simulink model "longitudinalMotion"  (R2023b)
settings: Solver=VariableStepAuto  StartTime=0.0  StopTime=30  FixedStep=0.01  RelTol=1e-3  AbsTol=1e-3  EnableMultiTasking=on
PreLoadFcn:
  | load terrainData
  | vehicleData
undefined symbols (not defined in the file or in its folder): FL, FR, RL, RR, slope
libraries: fl_lib x5, nesl_utility x4, sdl_lib x4, chassisTires_lib x1
settings Model: Creator=sseshadr  LastModifiedBy=mmedi
settings SolverCC: AutoScaleAbsTol=off  AlgebraicLoopSolver=TrustRegion
settings DataIOCC: LimitDataPoints=on  SaveFormat=Array  ReturnWorkspaceOutputs=off  SignalLoggingName=logsout_longitudinalMotion
settings OptimizationCC: ReuseModelBlockBuffer=off  LifeSpan=inf
settings DebuggingCC: UnconnectedInputMsg=warning  UnconnectedOutputMsg=warning  UnconnectedLineMsg=warning  SFUnexpectedBacktrackingDiag=warning  SFNoUnconditionalDefaultTransitionDiag=warning  SFExecutionAtInitializationDiag=none  ArithmeticOperatorsInVariantConditions=warning
settings HardwareCC: ProdBitPerPointer=32  ProdBitPerSizeT=32  ProdBitPerPtrDiffT=32  ProdLargestAtomicFloat=None  ProdIntDivRoundTo=Undefined  ProdEndianess=Unspecified  ProdWordSize=32  ProdHWDeviceType=32-bit Generic
settings ModelReferenceCC: EnableRefExpFcnMdlSchedulingChecks=on  PropagateSignalLabelsOutOfModel=off
settings SFSimCC: SimUseLocalCustomCode=off  CustomCodeUndefinedFunction=UseInterfaceOnly
settings RTWCC: RTWUseLocalCustomCode=off
settings CodeAppCC: StateflowObjectComments=on
settings GRTTargetCC: TargetLangStandard=C89/C90 (ANSI)
settings ConfigComp: CovMetricSettings=dw  CovSaveCumulativeToWorkspaceVar=on  CovSaveSingleToWorkspaceVar=on  CovExternalEMLEnable=off
settings SimscapeCC: SimscapeNormalizeSystem=off  SimscapeLogType=all  SimscapeLogSimulationStatistics=on  SimscapeLogToSDI=on  SimscapeLogName=simlog_longitudinalMotion  SimscapeLogDataHistory=10000

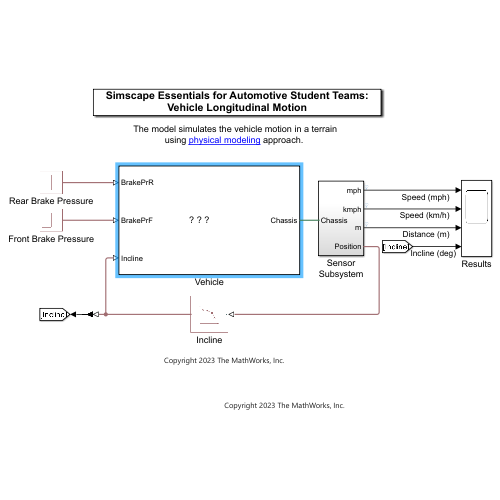
[thumbnail: Simulink's stored preview of the top-level diagram]
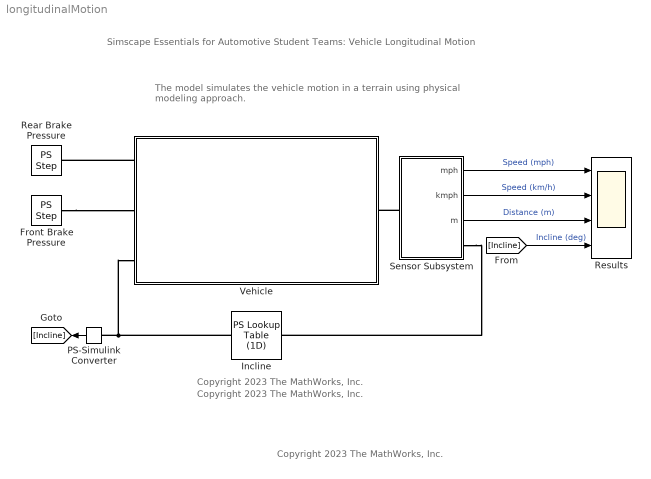
== system longitudinalMotion ==
  note: Copyright 2023 The MathWorks, Inc.
  note: Simscape Essentials for Automotive Student Teams: Vehicle Longitudinal Motion
  note: The model simulates the vehicle motion in a terrain using physical modeling approach.
  note: Copyright 2023 The MathWorks, Inc.
  note: Copyright 2023 The MathWorks, Inc.
  Front Brake Pressure : fl_lib/Physical Signals/Sources/PS Step  step_time=15 s  initial_value=0 N/m^2  final_value=brake.frontPressure N/(m^2)
  Incline : fl_lib/Physical Signals/Lookup Tables/PS Lookup Table (1D)  x=dist m  f=slope*1.2 rad  interp_method=simscape.enum.interpolation.linear  extrap_method=simscape.enum.extrapolation.linear
  PS-Simulink Converter : nesl_utility/PS-Simulink Converter  PhysicalDomain=network_engine_domain  SubClassName=ps_output  LeftPortType=input  RightPortType=output  PseudoPeriodic=off  Frequencies=[]  VectorFormat=inherit  Unit=deg  AffineConversion=off
  Rear Brake Pressure : fl_lib/Physical Signals/Sources/PS Step  step_time=12 s  initial_value=0 N/m^2  final_value=brake.rearPressure N/(m^2)
  Results : Scope  NumInputPorts=4
  Sensor Subsystem : Subsystem
  Vehicle : Subsystem
      mask Display: image('Images/vehicle.jpg'); % Use "Edit Image" on toolstrip to change.
  wires:
  Sensor Subsystem/1(mph) -> Results/1  "Speed (mph)"
  Sensor Subsystem/2(kmph) -> Results/2  "Speed (km/h)"
  Sensor Subsystem/3(m) -> Results/3  "Distance (m)"
  PS-Simulink Converter/1 -> [Incline]
  [Incline] -> Results/4  "Incline (deg)"
  connections:
  Sensor Subsystem/LConn1 -- Vehicle/RConn1
  Incline/RConn1 -- Vehicle/LConn3 -- PS-Simulink Converter/LConn1
  Sensor Subsystem/RConn1 -- Incline/LConn1
  Vehicle/LConn1 -- Rear Brake Pressure/RConn1
  Front Brake Pressure/RConn1 -- Vehicle/LConn2

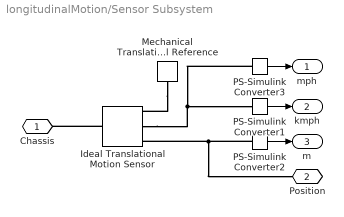
== system longitudinalMotion/Sensor Subsystem ==
  Ideal Translational Motion Sensor : fl_lib/Mechanical/Mechanical Sensors/Ideal Translational Motion Sensor  reference=foundation.enum.MeasurementReference.difference  acceleration_port=false  velocity_port=true  position_port=true  offset=0 m
  Mechanical Translational Reference : fl_lib/Mechanical/Translational Elements/Mechanical Translational Reference
  PS-Simulink Converter1 : nesl_utility/PS-Simulink Converter  PhysicalDomain=network_engine_domain  SubClassName=ps_output  LeftPortType=input  RightPortType=output  PseudoPeriodic=off  Frequencies=[]  VectorFormat=1-D array  Unit=km/hr  AffineConversion=off
  PS-Simulink Converter2 : nesl_utility/PS-Simulink Converter  PhysicalDomain=network_engine_domain  SubClassName=ps_output  LeftPortType=input  RightPortType=output  PseudoPeriodic=off  Frequencies=[]  VectorFormat=1-D array  Unit=1  AffineConversion=off
  PS-Simulink Converter3 : nesl_utility/PS-Simulink Converter  PhysicalDomain=network_engine_domain  SubClassName=ps_output  LeftPortType=input  RightPortType=output  PseudoPeriodic=off  Frequencies=[]  VectorFormat=1-D array  Unit=mph  AffineConversion=off
  Chassis : PMIOPort  Side=Left
  Position : PMIOPort  Port=2  Side=Right
  mph : Outport  VectorParamsAs1DForOutWhenUnconnected=off
  kmph : Outport  Port=2  VectorParamsAs1DForOutWhenUnconnected=off
  m : Outport  Port=3  VectorParamsAs1DForOutWhenUnconnected=off
  wires:
  PS-Simulink Converter1/1 -> kmph/1
  PS-Simulink Converter2/1 -> m/1
  PS-Simulink Converter3/1 -> mph/1
  connections:
  Mechanical Translational Reference/LConn1 -- Ideal Translational Motion Sensor/RConn1
  PS-Simulink Converter2/LConn1 -- Position/RConn1 -- Ideal Translational Motion Sensor/RConn3
  Ideal Translational Motion Sensor/RConn2 -- PS-Simulink Converter1/LConn1 -- PS-Simulink Converter3/LConn1
  Ideal Translational Motion Sensor/LConn1 -- Chassis/RConn1

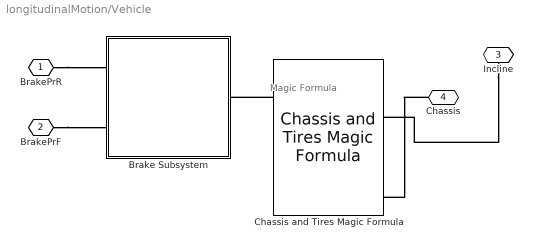
== system longitudinalMotion/Vehicle ==
  note: Magic Formula
  Brake Subsystem : Subsystem
  Chassis and Tires Magic Formula : chassisTires_lib/Chassis and Tires Magic Formula  SystemSampleTime=-1  VariantActivationTime=update diagram  AllowFlexibleInterface=on  Latency=0  AutoFrameSizeCalculation=off
  BrakePrR : PMIOPort  Side=Left
  BrakePrF : PMIOPort  Port=2  Side=Left
  Incline : PMIOPort  Port=3  Side=Left
  Chassis : PMIOPort  Port=4  Side=Right
  connections:
  Chassis/RConn1 -- Chassis and Tires Magic Formula/RConn3
  Incline/RConn1 -- Chassis and Tires Magic Formula/RConn1
  Chassis and Tires Magic Formula/LConn1 -- Brake Subsystem/RConn1
  BrakePrR/RConn1 -- Brake Subsystem/LConn1
  BrakePrF/RConn1 -- Brake Subsystem/LConn2

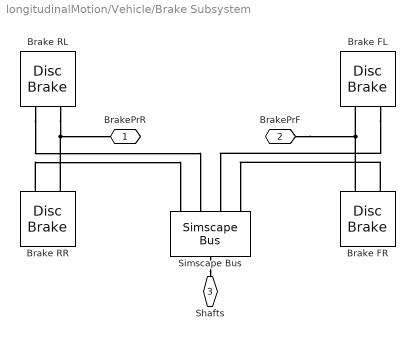
== system longitudinalMotion/Vehicle/Brake Subsystem ==
  Brake FL : sdl_lib/Brakes & Detents/Rotational/Disc Brake  r_mean=brake.padRadius mm  bore=brake.cylinderBore mm  n_pads=1  thermal_port=simscape.enum.thermaleffects.omit  mu_static=brake.sf  mu_coulomb=brake.cf  temperature_TLU=[280, 300, 320] K  mu_static_TLU=[.9, .8, .7]  mu_coulomb_TLU=[.8, .7, .6]  brkwy_vel=brake.frictionVel rad/s  visc_coef=brake.vfc N*m*s/rad  enable_faults=simscape.enum.onoff.off  faulted_pressure=0 bar  external_fault=simscape.enum.onoff.off  temporal_fault=simscape.enum.onoff.off  fault_time=5 s  report_fault=simscape.enum.assert.action.none  thermal_mass=50 kJ/K  temperature_specify=off  temperature_priority=High  temperature=300 K  temperature_nominal_specify=off  temperature_nominal_unit=K  temperature_nominal_value=1
  Brake FR : sdl_lib/Brakes & Detents/Rotational/Disc Brake  r_mean=brake.padRadius mm  bore=brake.cylinderBore mm  n_pads=1  thermal_port=simscape.enum.thermaleffects.omit  mu_static=brake.sf  mu_coulomb=brake.cf  temperature_TLU=[280, 300, 320] K  mu_static_TLU=[.9, .8, .7]  mu_coulomb_TLU=[.8, .7, .6]  brkwy_vel=brake.frictionVel rad/s  visc_coef=brake.vfc N*m*s/rad  enable_faults=simscape.enum.onoff.off  faulted_pressure=0 bar  external_fault=simscape.enum.onoff.off  temporal_fault=simscape.enum.onoff.off  fault_time=5 s  report_fault=simscape.enum.assert.action.none  thermal_mass=50 kJ/K  temperature_specify=off  temperature_priority=High  temperature=300 K  temperature_nominal_specify=off  temperature_nominal_unit=K  temperature_nominal_value=1
  Brake RL : sdl_lib/Brakes & Detents/Rotational/Disc Brake  r_mean=brake.padRadius mm  bore=brake.cylinderBore mm  n_pads=1  thermal_port=simscape.enum.thermaleffects.omit  mu_static=brake.sf  mu_coulomb=brake.cf  temperature_TLU=[280, 300, 320] K  mu_static_TLU=[.9, .8, .7]  mu_coulomb_TLU=[.8, .7, .6]  brkwy_vel=brake.frictionVel rad/s  visc_coef=brake.vfc N*m*s/rad  enable_faults=simscape.enum.onoff.off  faulted_pressure=0 bar  external_fault=simscape.enum.onoff.off  temporal_fault=simscape.enum.onoff.off  fault_time=5 s  report_fault=simscape.enum.assert.action.none  thermal_mass=50 kJ/K  temperature_specify=off  temperature_priority=High  temperature=300 K  temperature_nominal_specify=off  temperature_nominal_unit=K  temperature_nominal_value=1
  Brake RR : sdl_lib/Brakes & Detents/Rotational/Disc Brake  r_mean=brake.padRadius mm  bore=brake.cylinderBore mm  n_pads=1  thermal_port=simscape.enum.thermaleffects.omit  mu_static=brake.sf  mu_coulomb=brake.cf  temperature_TLU=[280, 300, 320] K  mu_static_TLU=[.9, .8, .7]  mu_coulomb_TLU=[.8, .7, .6]  brkwy_vel=brake.frictionVel rad/s  visc_coef=brake.vfc N*m*s/rad  enable_faults=simscape.enum.onoff.off  faulted_pressure=0 bar  external_fault=simscape.enum.onoff.off  temporal_fault=simscape.enum.onoff.off  fault_time=5 s  report_fault=simscape.enum.assert.action.none  thermal_mass=50 kJ/K  temperature_specify=off  temperature_priority=High  temperature=300 K  temperature_nominal_specify=off  temperature_nominal_unit=K  temperature_nominal_value=1
  Simscape Bus : SimscapeBus  HierarchyStrings=RR;RL;FL;FR
  BrakePrR : PMIOPort  Side=Left
  BrakePrF : PMIOPort  Port=2  Side=Left
  Shafts : PMIOPort  Port=3  Side=Right
  connections:
  BrakePrF/RConn1 -- Brake FR/LConn1 -- Brake FL/LConn1
  Brake RR/LConn1 -- Brake RL/LConn1 -- BrakePrR/RConn1
  Brake RR/LConn2 -- Simscape Bus/LConn1
  Brake FL/LConn2 -- Simscape Bus/LConn3
  Brake FR/LConn2 -- Simscape Bus/LConn4
  Simscape Bus/RConn1 -- Shafts/RConn1
  Brake RL/LConn2 -- Simscape Bus/LConn2
